simulink model "SoleModelNoDistrubance"  (R2019b)
settings: Solver=FixedStepAuto  StartTime=0.0  StopTime=6  FixedStep=0.001  RelTol=1e-3  AbsTol=1e-6
PreLoadFcn:
  | Kp =0.0614; Ki = 0.0723;
Description:
  | Engine Timing Model With Closed Loop Control
  | 
  | This example shows how to use triggered subsystems in Simulink(R) to model
  | engine timing, including a feedback controller. Different subsystems in the diagram
  | model the mathematical representation of various automotive systems, including
  | the following:
  | 
  | * Throttle and manifold
  | * Compression
  | * Combustion
  | * Vehicle dynamics
  | * Valve timing
  | * Controller
  | 
  | The valve timing subsystem generates a signal that triggers the Controller and
  | Compression subsystems twice per revolution of the crank (calculated from the
  | crank speed.) A speed set point (in rpm) from the Step block drives the simulation.
  | The controller calculates the necessary throttle angle based on the desired rpm
  | and the crank speed that is calculated by the vehicle dynamics. After you run
  | the simulation, the Scopes show the engine speed and the throttle angle
  | compared to the load torque.
settings Model: ExtModeTrigMode=oneshot  ExtModeArmWhenConnect=off  ExtModeAutoUpdateStatusClock=off  Creator=The MathWorks, Inc.  LastModifiedBy=Emanuel
settings SolverCC: AutoScaleAbsTol=off
settings DataIOCC: ExternalInput=[]  InitialState=[]  SaveFormat=Array  SaveOutput=off  SaveTime=off  ReturnWorkspaceOutputs=off  StateSaveName=x  TimeSaveName=t  OutputSaveName=y  SignalLoggingName=sldemo_enginewc_output
settings OptimizationCC: BlockReduction=off  ExpressionDepthLimit=2147483647  InitFltsAndDblsToZero=on  LifeSpan=inf  BufferReusableBoundary=off
settings DebuggingCC: SaveWithParameterizedLinksMsg=none  UnderspecifiedInitializationDetection=Classic  MergeDetectMultiDrivingBlocksExec=none  SignalResolutionControl=TryResolveAllWithWarning  MultiTaskDSMMsg=warning  MultiTaskCondExecSysMsg=none  SigSpecEnsureSampleTimeMsg=none  IntegerOverflowMsg=none  FcnCallInpInsideContextMsg=warning  BusObjectLabelMismatch=none  AllowSymbolicDim=off  StateNameClashWarn=warning  SFUnexpectedBacktrackingDiag=warning  SFNoUnconditionalDefaultTransitionDiag=warning  SFExecutionAtInitializationDiag=none  IntegerSaturationMsg=none  ArithmeticOperatorsInVariantConditions=warning
settings HardwareCC: ProdBitPerPointer=32  ProdBitPerSizeT=32  ProdBitPerPtrDiffT=32  ProdLargestAtomicFloat=None  ProdIntDivRoundTo=Undefined  ProdEndianess=Unspecified  ProdWordSize=32  ProdHWDeviceType=32-bit Generic
settings ModelReferenceCC: PropagateSignalLabelsOutOfModel=off
settings SFSimCC: SimUseLocalCustomCode=off  CustomCodeUndefinedFunction=UseInterfaceOnly
settings RTWCC: Description=Generic Real-Time Target  RTWUseLocalCustomCode=off
settings CodeAppCC: StateflowObjectComments=on
settings GRTTargetCC: TargetFcnLib=ansi_tfl_tmw.mat  TargetLangStandard=C89/C90 (ANSI)  GeneratePreprocessorConditionals=Disable all  CombineOutputUpdateFcns=off  GRTInterface=on
settings ConfigComp: CovMetricSettings=d  CovHtmlReporting=on  CovSaveCumulativeToWorkspaceVar=on  CovSaveSingleToWorkspaceVar=on  CovExternalEMLEnable=off

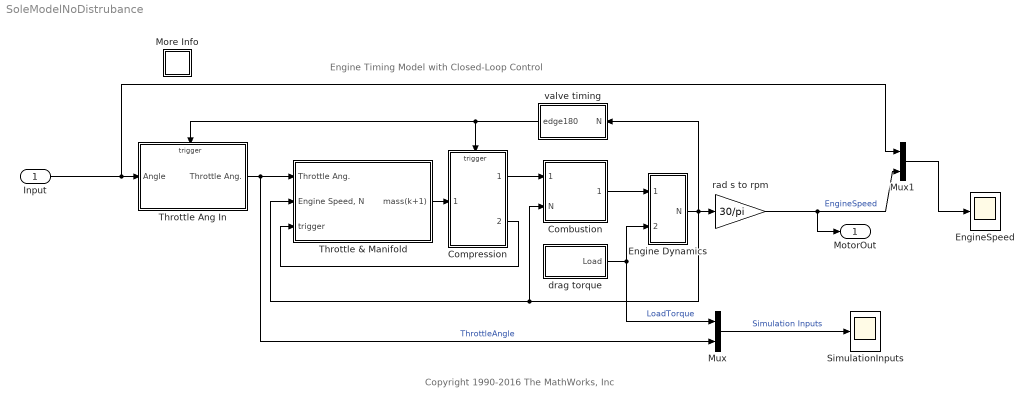
== system SoleModelNoDistrubance ==
  note: Engine Timing Model with Closed-Loop Control
  note: Copyright 1990-2016 The MathWorks, Inc
  Input : Inport
  Combustion : Subsystem
  Compression : Subsystem  TreatAsAtomicUnit=on
  Engine Dynamics : Subsystem
  EngineSpeed : Scope
  More Info : Subsystem
      settings: OpenFcn=showdemo(bdroot(gcb))
      mask Display: disp('?')
  Mux : Mux  Inputs=2
  Mux1 : Mux  Inputs=2
  SimulationInputs : Scope
  Throttle & Manifold : Subsystem
  Throttle Ang In : Subsystem  TreatAsAtomicUnit=on
  drag torque : Subsystem
  rad s to rpm : Gain  Gain=30/pi  SaturateOnIntegerOverflow=on  OutDataTypeStr=Inherit: Same as input  ParamDataTypeStr=Inherit: Same as input
  valve timing : Subsystem
  "MotorOut " : Outport
  wires:
  Input/1 -> Mux1/1, Throttle Ang In/1(Angle)
  drag torque/1(Load) -> Mux/1, Engine Dynamics/2(Tload)  "LoadTorque"
  Throttle Ang In/1(Throttle Ang.) -> Mux/2, Throttle & Manifold/1(Throttle Ang.)  "ThrottleAngle"
  Compression/1(mass(k)) -> Combustion/1(Air Charge)
  valve timing/1(edge180) -> Throttle Ang In/Trigger, Compression/Trigger
  Combustion/1(Torque) -> Engine Dynamics/1(Teng)
  Engine Dynamics/1(N) -> rad s to rpm/1, valve timing/1(N), Throttle & Manifold/2("Engine Speed, N"), Combustion/2(N)
  rad s to rpm/1 -> "MotorOut "/1, Mux1/2  "EngineSpeed"
  Mux/1 -> SimulationInputs/1  "Simulation Inputs"
  Throttle & Manifold/1(mass(k+1)) -> Compression/1(mass(k+1))
  Compression/2(trigger) -> Throttle & Manifold/3(trigger)
  Mux1/1 -> EngineSpeed/1

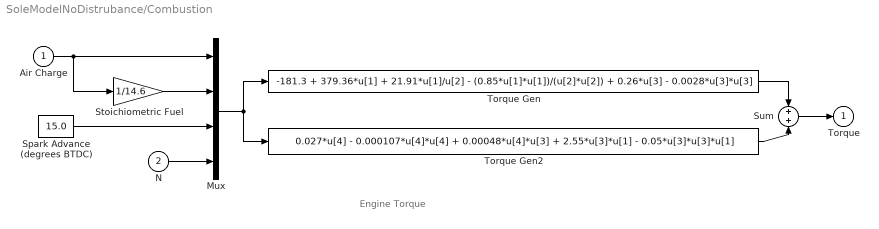
== system SoleModelNoDistrubance/Combustion ==
  note: Engine Torque
  Air Charge : Inport
  N : Inport  Port=2
  Mux : Mux
  Spark Advance (degrees BTDC) : Constant  Value=15.0
  Stoichiometric Fuel : Gain  Gain=1/14.6  SaturateOnIntegerOverflow=on  OutDataTypeStr=Inherit: Same as input  ParamDataTypeStr=Inherit: Same as input
  Sum : Sum  SaturateOnIntegerOverflow=on  InputSameDT=on  OutDataTypeStr=Inherit: Same as first input
  Torque Gen : Fcn  Expr=-181.3 + 379.36*u[1] + 21.91*u[1]/u[2] - (0.85*u[1]*u[1])/(u[2]*u[2]) + 0.26*u[3] - 0.0028*u[3]*u[3]
  Torque Gen2 : Fcn  Expr=0.027*u[4] - 0.000107*u[4]*u[4] + 0.00048*u[4]*u[3] + 2.55*u[3]*u[1] - 0.05*u[3]*u[3]*u[1]
  Torque : Outport  InitialOutput=0
  wires:
  Stoichiometric Fuel/1 -> Mux/2
  Spark Advance (degrees BTDC)/1 -> Mux/3
  N/1 -> Mux/4
  Air Charge/1 -> Stoichiometric Fuel/1, Mux/1
  Mux/1 -> Torque Gen/1, Torque Gen2/1
  Torque Gen2/1 -> Sum/2
  Torque Gen/1 -> Sum/1
  Sum/1 -> Torque/1

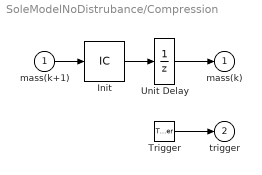
== system SoleModelNoDistrubance/Compression ==
  mass(k+1) : Inport
  Trigger : TriggerPort  TriggerType=either  VariantControl=Variant  ShowOutputPort=on
  Init : InitialCondition  Value=0.152
  Unit Delay : UnitDelay  InitialCondition=0.152  SampleTime=-1  HasFrameUpgradeWarning=on
  mass(k) : Outport  InitialOutput=0.152
  trigger : Outport  Port=2  InitialOutput=-1
  wires:
  Init/1 -> Unit Delay/1
  mass(k+1)/1 -> Init/1
  Unit Delay/1 -> mass(k)/1
  Trigger/1 -> trigger/1

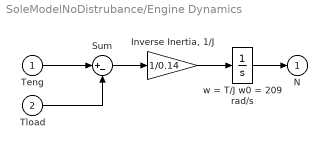
== system SoleModelNoDistrubance/Engine Dynamics ==
  Teng : Inport
  Tload : Inport  Port=2
  "Inverse Inertia, 1/J" : Gain  Gain=1/0.14  SaturateOnIntegerOverflow=on  OutDataTypeStr=Inherit: Same as input  ParamDataTypeStr=Inherit: Same as input
  Sum : Sum  Inputs=|+-  SaturateOnIntegerOverflow=on  InputSameDT=on  OutDataTypeStr=Inherit: Same as first input
  w = T/J w0 = 209 rad/s : Integrator  InitialCondition=209.48
  N : Outport  InitialOutput=0
  wires:
  "Inverse Inertia, 1/J"/1 -> w = T/J w0 = 209 rad/s/1
  w = T/J w0 = 209 rad/s/1 -> N/1
  Sum/1 -> "Inverse Inertia, 1/J"/1
  Teng/1 -> Sum/1
  Tload/1 -> Sum/2

== system SoleModelNoDistrubance/More Info ==

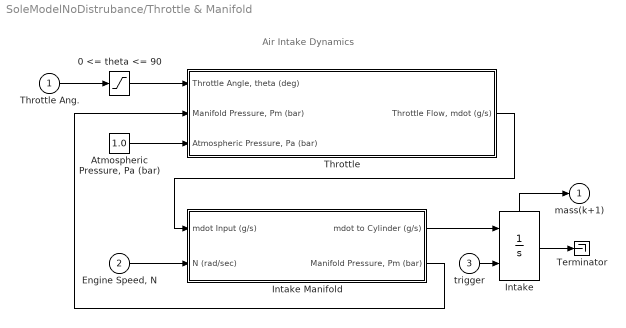
== system SoleModelNoDistrubance/Throttle & Manifold ==
  note: Air Intake Dynamics
  Throttle Ang. : Inport
  "Engine Speed, N" : Inport  Port=2
  trigger : Inport  Port=3
  0 <= theta <= 90 : Saturate  UpperLimit=90  LowerLimit=0
  "Atmospheric Pressure, Pa (bar)" : Constant  Value=1.0
  Intake : Integrator  ExternalReset=either  ShowStatePort=on
  Intake Manifold : Subsystem
  Terminator : Terminator
  Throttle : Subsystem
  mass(k+1) : Outport  InitialOutput=0
  wires:
  0 <= theta <= 90/1 -> Throttle/1("Throttle Angle, theta (deg)")
  Throttle Ang./1 -> 0 <= theta <= 90/1
  Throttle/1("Throttle Flow, mdot (g/s)") -> Intake Manifold/1(mdot Input (g/s))
  "Engine Speed, N"/1 -> Intake Manifold/2(N (rad/sec))
  Intake Manifold/2("Manifold Pressure, Pm (bar)") -> Throttle/2("Manifold Pressure, Pm (bar)")
  Intake Manifold/1(mdot to Cylinder (g/s)) -> Intake/1
  "Atmospheric Pressure, Pa (bar)"/1 -> Throttle/3("Atmospheric Pressure, Pa (bar) ")
  Intake/State -> mass(k+1)/1
  trigger/1 -> Intake/2
  Intake/1 -> Terminator/1

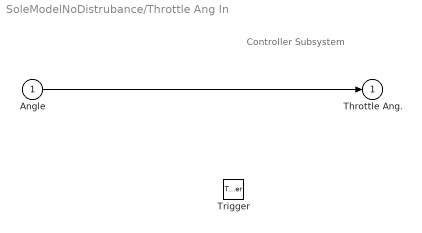
== system SoleModelNoDistrubance/Throttle Ang In ==
  note: Controller Subsystem
  Angle : Inport
  Trigger : TriggerPort  TriggerType=either  VariantControl=Variant
  Throttle Ang. : Outport  InitialOutput=8.973
  wires:
  Angle/1 -> Throttle Ang./1

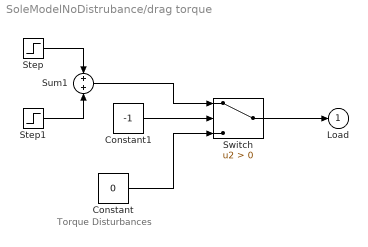
== system SoleModelNoDistrubance/drag torque ==
  note: Torque Disturbances
  Constant : Constant  Value=0
  Constant1 : Constant  Value=-1
  Step : Step  Time=2  Before=25  After=20  SampleTime=0
  Step1 : Step  Time=8  After=5  SampleTime=0
  Sum1 : Sum  SaturateOnIntegerOverflow=on  InputSameDT=on  OutDataTypeStr=Inherit: Same as first input
  Switch : Switch  Criteria=u2 > Threshold
  Load : Outport  InitialOutput=0
  wires:
  Sum1/1 -> Switch/1
  Step/1 -> Sum1/1
  Step1/1 -> Sum1/2
  Switch/1 -> Load/1
  Constant/1 -> Switch/3
  Constant1/1 -> Switch/2

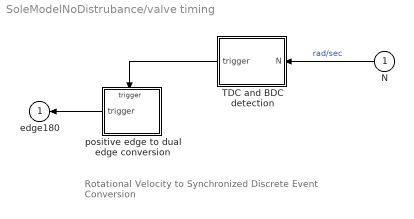
== system SoleModelNoDistrubance/valve timing ==
  note: Rotational Velocity to Synchronized
      | Discrete Event Conversion
  N : Inport
  TDC and BDC detection : Subsystem
  positive edge to dual edge conversion : Subsystem  TreatAsAtomicUnit=on
  edge180 : Outport  InitialOutput=-1
  wires:
  TDC and BDC detection/1(trigger) -> positive edge to dual edge conversion/Trigger
  positive edge to dual edge conversion/1(trigger) -> edge180/1
  N/1 -> TDC and BDC detection/1(N)  "rad/sec"

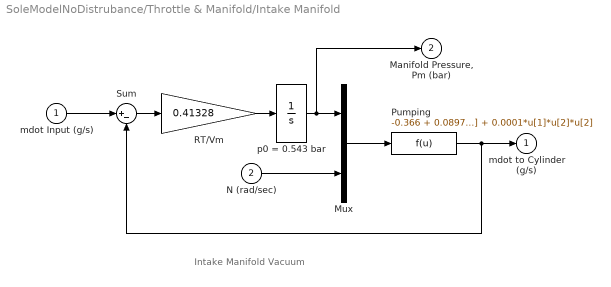
== system SoleModelNoDistrubance/Throttle & Manifold/Intake Manifold ==
  note: Intake Manifold Vacuum
  mdot Input (g/s) : Inport
  N (rad/sec) : Inport  Port=2
  Mux : Mux  Inputs=2
  Pumping : Fcn  Expr=-0.366 + 0.08979*u[1]*u[2] - 0.0337*u[2]*u[1]*u[1] + 0.0001*u[1]*u[2]*u[2]
  RT/Vm : Gain  Gain=0.41328  SaturateOnIntegerOverflow=on  OutDataTypeStr=Inherit: Same as input  ParamDataTypeStr=Inherit: Same as input
  Sum : Sum  Inputs=|+-  SaturateOnIntegerOverflow=on  InputSameDT=on  OutDataTypeStr=Inherit: Same as first input
  p0 = 0.543 bar : Integrator  InitialCondition=.543
  mdot to Cylinder (g/s) : Outport  InitialOutput=0
  "Manifold Pressure, Pm (bar)" : Outport  Port=2  InitialOutput=0
  wires:
  mdot Input (g/s)/1 -> Sum/1
  RT/Vm/1 -> p0 = 0.543 bar/1
  N (rad/sec)/1 -> Mux/2
  Mux/1 -> Pumping/1
  p0 = 0.543 bar/1 -> Mux/1, "Manifold Pressure, Pm (bar)"/1
  Sum/1 -> RT/Vm/1
  Pumping/1 -> Sum/2, mdot to Cylinder (g/s)/1

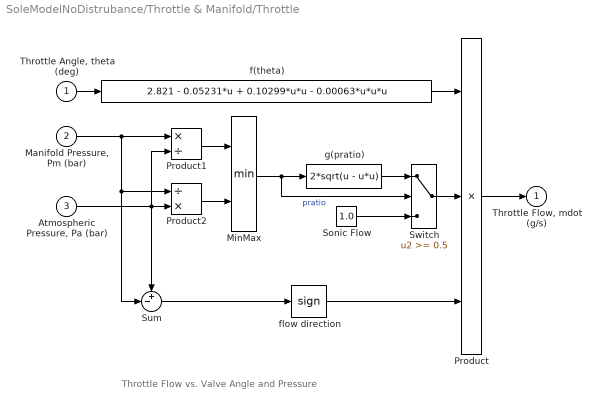
== system SoleModelNoDistrubance/Throttle & Manifold/Throttle ==
  note: Throttle Flow vs. Valve Angle and Pressure
  "Throttle Angle, theta (deg)" : Inport
  "Manifold Pressure, Pm (bar)" : Inport  Port=2
  "Atmospheric Pressure, Pa (bar) " : Inport  Port=3
  MinMax : MinMax  Inputs=2  SaturateOnIntegerOverflow=on  InputSameDT=on
  Product : Product  Inputs=3  SaturateOnIntegerOverflow=on  RndMeth=Zero  InputSameDT=on  OutDataTypeStr=Inherit: Same as first input
  Product1 : Product  Inputs=*/  SaturateOnIntegerOverflow=on  RndMeth=Zero  InputSameDT=on  OutDataTypeStr=Inherit: Same as first input
  Product2 : Product  Inputs=/*  SaturateOnIntegerOverflow=on  RndMeth=Zero  InputSameDT=on  OutDataTypeStr=Inherit: Same as first input
  "Sonic Flow " : Constant  Value=1.0
  Sum : Sum  Inputs=+-|  SaturateOnIntegerOverflow=on  InputSameDT=on  OutDataTypeStr=Inherit: Same as first input
  Switch : Switch  Threshold=0.5  SaturateOnIntegerOverflow=on  InputSameDT=on
  f(theta) : Fcn  Expr=2.821 - 0.05231*u + 0.10299*u*u - 0.00063*u*u*u
  flow direction : Signum
  g(pratio) : Fcn  Expr=2*sqrt(u - u*u)
  "Throttle Flow, mdot (g/s)" : Outport  InitialOutput=0
  wires:
  "Manifold Pressure, Pm (bar)"/1 -> Sum/2, Product2/1, Product1/1
  Product2/1 -> MinMax/2
  Product1/1 -> MinMax/1
  "Atmospheric Pressure, Pa (bar) "/1 -> Sum/1, Product2/2, Product1/2
  g(pratio)/1 -> Switch/1
  "Sonic Flow "/1 -> Switch/3
  Switch/1 -> Product/2
  flow direction/1 -> Product/3
  Sum/1 -> flow direction/1
  MinMax/1 -> Switch/2, g(pratio)/1  "pratio"
  "Throttle Angle, theta (deg)"/1 -> f(theta)/1
  Product/1 -> "Throttle Flow, mdot (g/s)"/1
  f(theta)/1 -> Product/1

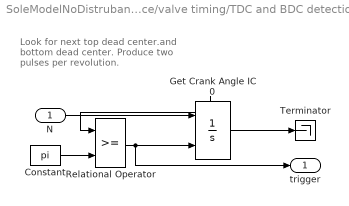
== system SoleModelNoDistrubance/valve timing/TDC and BDC detection ==
  note: Look for next top dead center.and
      | bottom dead center.
      | Produce two pulses per revolution.
  N : Inport
  Constant : Constant  Value=pi
  Get Crank Angle IC 0 : Integrator  ExternalReset=rising  ShowStatePort=on
  Relational Operator : RelationalOperator  OutDataTypeStr=boolean  RndMeth=Nearest  InputSameDT=on
  Terminator : Terminator
  trigger : Outport  InitialOutput=0
  wires:
  N/1 -> Get Crank Angle IC 0/1
  Relational Operator/1 -> trigger/1, Get Crank Angle IC 0/2
  Constant/1 -> Relational Operator/2
  Get Crank Angle IC 0/State -> Relational Operator/1
  Get Crank Angle IC 0/1 -> Terminator/1

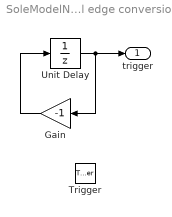
== system SoleModelNoDistrubance/valve timing/positive edge to dual edge conversion ==
  Trigger : TriggerPort  VariantControl=Variant
  Gain : Gain  Gain=-1  SaturateOnIntegerOverflow=on  OutDataTypeStr=Inherit: Same as input  ParamDataTypeStr=Inherit: Same as input
  Unit Delay : UnitDelay  InitialCondition=1  SampleTime=-1  HasFrameUpgradeWarning=on
  trigger : Outport  InitialOutput=-1
  wires:
  Gain/1 -> Unit Delay/1
  Unit Delay/1 -> trigger/1, Gain/1
